simulink model "Rate_Meas_RS232_HFC_1P"  (Simulink 7.8)
settings: Solver=VariableStepDiscrete  StartTime=0.0  StopTime=Inf  FixedStep=Ts/4  RelTol=1e-3
PreLoadFcn:
  | clear all;
  | close all;
  | clc;
  | 
  | Ts = 0.01;          % clk (period)
  | Ns =  1;
StartFcn:
  | clc;
  | close all;
  | 
  | Ns =  200;      % Characters to Tx and to Rx
  | minV = 0;       %  minimum data value
  | maxV = 255;       %  minimum data value
  | Tx_array = randi([minV maxV], 1, Ns, 'uint8');
  | Rx_array = randi([minV maxV], 1, Ns, 'uint8');
  | 
  | 
  | %
  | %   RS232 port initialization
  | %
  | PORTNAME = 'COM56';
  | fprintf('\nOpening RS232 port %s ...... ', PORTNAME);
  | s2 = serial(PORTNAME,'BaudRate',9600,'Parity','none','DataBits',8);
  | set(s2, 'FlowControl', 'none');
  | set(s2, 'InputBufferSize', 64);
  | set(s2, 'OutputBufferSize', 1);
  | fopen(s2);
  | s1.RecordDetail = 'verbose';
  | s1.RecordName = 'uart2.txt';
  | record(s2,'on')
  | fprintf('\nRS232 port %s activated\n', PORTNAME);
  | 
  | b2o_s2 = uint8(0);
  | d2o_s2 = uint8(0);
  | b2r_s2 = uint8(0);
  | d2r_s2 = uint8(0);
  | rts_s2 = uint8(0);
  | cts_s2 = uint8(0);
  | 
  | 
  | ts = tic;
StopFcn:
  | e_time = toc(ts);
  | 
  | %
  | %   RS232 ports release
  | %
  | disp(' ');
  | disp('Deactivating RS232 port ......');
  | 
  | fclose(s2)
  | delete(s2)
  | clear s2
  | 
  | fprintf('RS232 port %s deactivated\n', PORTNAME);
  | 
  | if Tx_array == Rx_array
  |   disp('Data exchange without errors');
  |   fprintf('\nData Rate = %4.2f Bps\n', Ns/e_time);
  | else
  |    Ne = sum((Tx_array - Rx_array) ~= 0);
  |    fprintf('\nData exchange with %d errors in %d data charactes\n\n', Ne, Ns);
  | end
libraries: simulink x1
settings Model: Creator=theodore  LastModifiedBy=theodore
settings DebuggingCC: SolverPrmCheckMsg=none
settings CodeAppCC: CustomSymbolStrType=$N$R$M_T

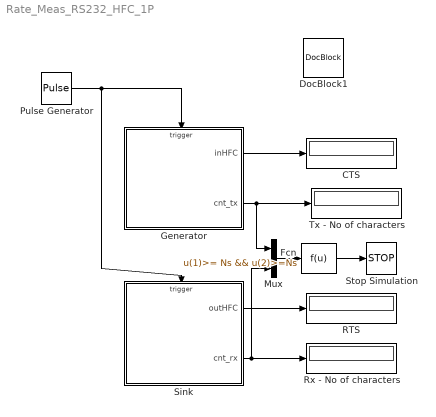
== system Rate_Meas_RS232_HFC_1P ==
  CTS : Display
  DocBlock1 : simulink/Model-Wide Utilities/DocBlock  DocumentType=Text
      content=|
      | Generator using RTS  and Sink using CTS
  Fcn : Fcn  Expr=u(1)>= Ns && u(2)>=Ns
  Generator : Stateflow chart  TreatAsAtomicUnit=on
  Mux : Mux  Inputs=2
  Pulse Generator : DiscretePulseGenerator  PulseType=Time based  Period=Ts  PulseWidth=50
  RTS : Display
  Rx - No of characters : Display
  Sink : Stateflow chart  TreatAsAtomicUnit=on
  Stop Simulation : Stop
  Tx - No of characters : Display
  wires:
  Pulse Generator/1 -> Generator/Trigger, Sink/Trigger
  Sink/2(cnt_rx) -> Rx - No of characters/1, Mux/2
  Sink/1(outHFC) -> RTS/1
  Generator/1(inHFC) -> CTS/1
  Generator/2(cnt_tx) -> Tx - No of characters/1, Mux/1
  Fcn/1 -> Stop Simulation/1
  Mux/1 -> Fcn/1

== stateflow chart Sink ==
  state RxState
    en: ml('DIn_2');
    Val_rx = ml.d2r_s2;
    cnt_rx = cnt_rx + 1;
    ml.Rx_array[cnt_rx] = Val_rx;
  state IniState
  IniState -> (junction 5) : {ml('B2R_2'); }
  RxState -> IniState
  (default) -> IniState : {cnt_rx = 0;
      | ml.rts_s2 = 1;
      | outHFC = 1;
      | ml('RTS_2');}
  (junction 5) -> IniState [order 1] : [ml.b2r_s2 == 0 ]
  (junction 5) -> RxState [order 2]
  data: outHFC output double; Val_rx local uint8; cnt_rx output double; LBstatus_rx local double =0
  events: CLK input RISING_EDGE_EVENT

== stateflow chart Generator ==
  state Dcalc
    en: ml('CTS_2');
    LBstatus_tx = ml.cts_s2;
    inHFC = LBstatus_tx;
  state IniState
    ml('CTS_2');
    LBstatus_tx = ml.cts_s2;
    inHFC = LBstatus_tx;
  state TxState
    en: cnt_tx = cnt_tx + 1;
    Val_tx = ml.Tx_array[cnt_tx];
    ml.d2o_s2 = Val_tx;
    ml('DOut_2');
  state Idle
  (junction 23) -> TxState [order 1] : [LBstatus_tx  ~= 0 ]
  (junction 22) -> Dcalc [order 2]
  (default) -> IniState : {cnt_tx = 0;}
  (junction 22) -> IniState [order 1] : [ml.b2o_s2 > 0 || LBstatus_tx == 0]
  TxState -> (junction 24)
  IniState -> (junction 22) : {ml('B2O_2'); }
  Dcalc -> (junction 23)
  (junction 23) -> Dcalc [order 2]
  (junction 24) -> Idle [order 1] : [cnt_tx == ml.Ns]
  (junction 24) -> IniState [order 2]
  data: inHFC output double; cnt_tx output double; Val_tx local uint8; LBstatus_tx local double =0
  events: CLK input RISING_EDGE_EVENT
